simulink model "VCU_SW"  (R2020b)
settings: Solver=FixedStepDiscrete  StartTime=0.0  StopTime=inf  FixedStep=1e-2  RelTol=1e-3
PreLoadFcn:
  | RTWConfigurationCB('preloadfcn', bdroot);
InitFcn:
  | loadvar_ttc500
undefined symbols (not defined in the file): BrkPedalTypes, CabMovModeTypes, cFuseTempSensAcc_X, cFuseTempSensAcc_Y, cFuseTempSensVal_X, cFuseTempSensVal_Y, cTMSTempSensVal_X, cTMSTempSensVal_Y, cTransferCaseSpeedRatio, diag_state, DoorsPositionTypes, dP_filter_Y, DriverOccClassSystemTypes, ErrorValueTypes, fatal_error_callback, IO_ADC_NO_RANGE, LadderStatusTypes, pAnalogCabRotSensAcc, pAnalogCabRotSensMaxVolt, pAnalogCabRotSensMinVolt, pAnalogCabRotSensRange, pAnalogCabRotSensZeroVolt, pBrkActivePress, pCabTiltSensAcc, pCabTiltSensMaxCur, pCabTiltSensMinCur, pDistanceCorrection, pECANManual_BPNEnable, pECANManual_BPNEnabler_Flag, pFilterSensAccRes, pHDirMaxDiffFrq, pHDirSensHighLvl, pHDirSensLowLvl, pMainGearRatio, pMaxFilterSensRes, pMaxFirstPedalSensValue, pMaxFuseTempSensRes, pMaxPressLoss, pMaxPressSensCurrent, pMaxPressValue, pMaxPressValueHydMotAndPump, pMaxPressValueParkDrain, pMaxSecondPedalSensValue, pMaxTempSensVoltage, pMaxTempValue, pMaxTMSTempSensRes, pMinFilterSensRes, pMinFirstPedalSensValue, pMinFuseTempSensRes, pMinPressLoss, pMinPressSensCurrent, pMinPressValue, pMinSecondPedalSensValue, pMinTempSensVoltage, pMinTempValue, pMinTMSTempSensRes, pMotorRingTeethNum, pPedalSensAccuracyPct, pPedalSensAccuracyVolt, pPressLossTreshhold ... (+20)
libraries: TTlibrary x270, canmsglib x127, simulink x88
(part 15 of 17)

== system VCU_SW/InputLayer/InputNetwork/InputCCAN/CCAN100msecProc1/CabMov buttons processing/callTiltFcn/setAutoTiltBut ==
  setAutoTiltBut : TriggerPort  TriggerType=function-call  IsSimulinkFunction=on  FunctionName=setAutoTiltBut  FunctionVisibility=scoped  VariantControl=(inherit)
  Data Store Write1 : DataStoreWrite  DataStoreName=InputFunctionsData  DataStoreElements=InputFunctionsData.stabBut
  Data Store Write2 : DataStoreWrite  DataStoreName=InputFunctionsData  DataStoreElements=InputFunctionsData.returnBut
  Enumerated Constant : simulink/Sources/Enumerated Constant  OutDataTypeStr=Enum: CabMovModeTypes  Value=CabMovModeTypes.CAB_TILT_RETURN  SampleTime=inf
  Enumerated Constant1 : simulink/Sources/Enumerated Constant  OutDataTypeStr=Enum: CabMovModeTypes  Value=CabMovModeTypes.CAB_TILT_STAB  SampleTime=inf
  Enumerated Constant2 : simulink/Sources/Enumerated Constant  OutDataTypeStr=Enum: StateModeTypes  Value=StateModeTypes.STT_DISABLE  SampleTime=inf
  Enumerated Constant3 : simulink/Sources/Enumerated Constant  OutDataTypeStr=Enum: StateModeTypes  Value=StateModeTypes.STT_ENABLE  SampleTime=inf
  Enumerated Constant4 : simulink/Sources/Enumerated Constant  OutDataTypeStr=Enum: StateModeTypes  Value=StateModeTypes.STT_DISABLE  SampleTime=inf
  Enumerated Constant5 : simulink/Sources/Enumerated Constant  OutDataTypeStr=Enum: StateModeTypes  Value=StateModeTypes.STT_ENABLE  SampleTime=inf
  Multiport Switch : MultiPortSwitch  DataPortOrder=Zero-based contiguous  Inputs=2  zeroidx=on
  Multiport Switch1 : MultiPortSwitch  DataPortOrder=Zero-based contiguous  Inputs=2  zeroidx=on
  Relational Operator : RelationalOperator  Operator===  OutDataTypeStr=boolean  RndMeth=Simplest
  Relational Operator1 : RelationalOperator  Operator===  OutDataTypeStr=boolean  RndMeth=Simplest
  state : ArgIn  OutDataTypeStr=Enum: CabMovModeTypes  ArgumentName=state
  wires:
  Multiport Switch1/1 -> Data Store Write1/1
  Enumerated Constant5/1 -> Multiport Switch1/3
  Enumerated Constant4/1 -> Multiport Switch1/2
  Enumerated Constant2/1 -> Multiport Switch/2
  Enumerated Constant3/1 -> Multiport Switch/3
  Multiport Switch/1 -> Data Store Write2/1
  Relational Operator1/1 -> Multiport Switch1/1
  Enumerated Constant1/1 -> Relational Operator1/2
  Relational Operator/1 -> Multiport Switch/1
  Enumerated Constant/1 -> Relational Operator/2
  state/1 -> Relational Operator/1, Relational Operator1/1

== system VCU_SW/InputLayer/InputNetwork/InputCCAN/CCAN100msecProc1/CabMov buttons processing/callTiltFcn/setTiltBut ==
  setTiltBut : TriggerPort  TriggerType=function-call  IsSimulinkFunction=on  FunctionName=setTiltBut  FunctionVisibility=scoped  VariantControl=(inherit)
  Data Store Read1 : DataStoreRead  DataStoreName=InputNetworkData  DataStoreElements=InputNetworkData.CCAN.BJM1.But3CabPitchFwd#InputNetworkData.CCAN.BJM1.But4CabPitchBckwd#InputNetworkData.CCAN.BJM1.But2CabRollLeft#InputNetworkData.CCAN.BJM1.But1CabRollRight
  Data Store Write1 : DataStoreWrite  DataStoreName=InputFunctionsData  DataStoreElements=InputFunctionsData.pitchFwdBut#InputFunctionsData.pitchBckwdBut#InputFunctionsData.rollLeftBut#InputFunctionsData.rollRightBut
  MATLAB Function : MATLAB Function  TreatAsAtomicUnit=on
  state : ArgIn  OutDataTypeStr=Enum: CabMovModeTypes  ArgumentName=state
  wires:
  state/1 -> MATLAB Function/1(state)
  MATLAB Function/1(pitchFwd) -> Data Store Write1/1
  MATLAB Function/2(pitchBckwd) -> Data Store Write1/2
  Data Store Read1/1 -> MATLAB Function/2(FwdBut)
  Data Store Read1/2 -> MATLAB Function/3(BckwdBut)
  Data Store Read1/3 -> MATLAB Function/4(LeftBut)
  Data Store Read1/4 -> MATLAB Function/5(RightBut)
  MATLAB Function/3(rollLeft) -> Data Store Write1/3
  MATLAB Function/4(rollRight) -> Data Store Write1/4

== system VCU_SW/InputLayer/InputNetwork/InputCCAN/CCAN100msecProc1/CabMov buttons processing/callTiltFcn/tiltReturnAchieved ==
  tiltReturnAchieved : TriggerPort  TriggerType=function-call  IsSimulinkFunction=on  FunctionName=tiltReturnAchieved  FunctionVisibility=scoped  VariantControl=(inherit)
  Constant3 : Constant  Value=pTiltAngleThres
  Constant4 : Constant  Value=pTiltAngleThres
  Data Store Read8 : DataStoreRead  DataStoreName=CabineControllerData  DataStoreElements=CabineControllerData.cabRollHullRef
  Data Store Read9 : DataStoreRead  DataStoreName=CabineControllerData  DataStoreElements=CabineControllerData.cabPitchHullRef
  OR3 : Logic  AllPortsSameDT=off  OutDataTypeStr=boolean
  Relational Operator11 : RelationalOperator  Operator=<=  OutDataTypeStr=boolean  RndMeth=Simplest
  Relational Operator9 : RelationalOperator  Operator=<=  OutDataTypeStr=boolean  RndMeth=Simplest
  result : ArgOut  OutDataTypeStr=boolean  ArgumentName=result
  wires:
  Constant3/1 -> Relational Operator9/2
  Data Store Read9/1 -> Relational Operator9/1
  Constant4/1 -> Relational Operator11/2
  OR3/1 -> result/1
  Relational Operator9/1 -> OR3/1
  Relational Operator11/1 -> OR3/2
  Data Store Read8/1 -> Relational Operator11/1

== matlab function VCU_SW/InputLayer/InputNetwork/InputDiagCAN/GetDiagCAN10msec/MATLAB Function ==
  data: ReadUDSmsgFlag output
function  ReadUDSmsgFlag = UDSClientFcn()

persistent flag

serviceSts = getUDSMsgSts(); 
if serviceSts == uint16(0)
    parsingUDSMsg();
    getWriteMsg();
    flag = true;
else
    flag = false;
end

ReadUDSmsgFlag = flag;

end

== matlab function VCU_SW/InputLayer/InputNetwork/InputDiagCAN/GetDiagCAN10msec/Simulink Function2/MATLAB Function2 ==
  data: UDSStruct data_store_memory
function getWriteUdsMsgFcn()

global UDSStruct

persistent flag

if UDSStruct.Service_id == uint8(hex2dec('2E')) && UDSStruct.sucReadFlag == true
    flag = true;
    if UDSStruct.DataIdentifier == uint16(0xB001)
        UDSStruct.TransPumpVolumeMax = uint16(UDSStruct.DataRecord);        
    elseif UDSStruct.DataIdentifier == uint16(0xB002)
        UDSStruct.TransMotorVolumeMin = uint16(UDSStruct.DataRecord);  
    elseif UDSStruct.DataIdentifier == uint16(0xB003)
        UDSStruct.AccelerationPedalMaxEngSpd = uint16(UDSStruct.DataRecord);
    elseif UDSStruct.DataIdentifier == uint16(0xB004)
        UDSStruct.AccelerationPedalMinEngSpd = uint16(UDSStruct.DataRecord);
    elseif UDSStruct.DataIdentifier == uint16(0xB101)
        UDSStruct.EngineSpeedMax = uint16(UDSStruct.DataRecord);
    elseif UDSStruct.DataIdentifier == uint16(0xB102)
        UDSStruct.EngineSpeedMin = uint16(UDSStruct.DataRecord);    
    else
        flag = false; 
    end
else
    flag = false; 
end

UDSStruct.WtiteUDSmsgFlag = flag; 

end

== matlab function VCU_SW/InputLayer/Simulink Function2/MATLAB Function ==
  data: volt input; state output; treshold input
function state = conv(volt, treshold)

if volt > treshold
    state = StateModeTypes.STT_ENABLE;
else
    state = StateModeTypes.STT_DISABLE;
end

end

== matlab function VCU_SW/OutputLayer/OutputNetwork/OutputDiagCAN + Logger/exLogger/MATLAB Function6 ==
  data: input input; value output
function value = fcn(input)

if input == StateModeTypes.STT_DISABLE
    value = uint8(0);
elseif input == StateModeTypes.STT_ENABLE
    value = uint8(1);
else
    value = uint8(0);
end

== matlab function VCU_SW/InputLayer/InputNetwork/InputCCAN/CCAN100msecProc1/CabMov buttons processing/MATLAB Function ==
function buttProcCaller()
    
    rotState = callRotFcn();
    callTiltFcn(rotState);
    
end

== matlab function VCU_SW/OutputLayer/OutputNetwork/OutputDiagCAN + Logger/SetDiagCAN10msec/MATLAB Function ==
  data: flag input
function getUDSmsgFcn(flag)
 
if flag 
    getUDSMsg();
end

end

== matlab function VCU_SW/ServerFcn/convINint1/MATLAB Function2 ==
  data: x input; y output
function y = fcn(x)

y = int16(x);

end

== matlab function VCU_SW/ServerFcn/convAIResistanceData/MATLAB Function ==
  data: inpValue input; outValue output; errorSts input
function outValue = convResValFcn(inpValue, errorSts)

if errorSts == uint16(0)
    %outValue = uint32(inpValue*single(1000));
    outValue = inpValue;
else
    outValue = uint32(ErrorValueTypes.RESISTANSE_ERROR_VALUE);
end

end

== matlab function VCU_SW/InputLayer/InputNetwork/InputCCAN/CCAN100msecProc1/CabMov buttons processing/callRotFcn/RotFcn ==
  data: rotState output; rotReturnTrigger input; manualRotReq input
function rotState = RotFcn(rotReturnTrigger, manualRotReq)

    persistent state
        if isempty(state)
            state = CabMovModeTypes.CAB_FIXED;
            setReturnBut(StateModeTypes.STT_DISABLE);
        end

    switch state
    
        case CabMovModeTypes.CAB_FIXED
            %Первый приоритет - вращение вручную
            if manualRotReq
                state = CabMovModeTypes.CAB_ROTATION;
            elseif rotReturnTrigger && ~rotReturnAchieved()
            %Второй приоритет - автоматический возврат
                state = CabMovModeTypes.CAB_ROTATION_RETURN;
                setReturnBut(StateModeTypes.STT_ENABLE);
            end
            
        case CabMovModeTypes.CAB_ROTATION
            if ~manualRotReq
                state = CabMovModeTypes.CAB_FIXED;
            end
            
        case CabMovModeTypes.CAB_ROTATION_RETURN
            %Выход т.к. джойстик приоритетней
            if manualRotReq
                state = CabMovModeTypes.CAB_ROTATION;
                setReturnBut(StateModeTypes.STT_DISABLE);
            %Выход т.к. закончили возврат либо повторно нажали на кнопку
            elseif rotReturnAchieved() || rotReturnTrigger
                state = CabMovModeTypes.CAB_FIXED;
                setReturnBut(StateModeTypes.STT_DISABLE);
            end
            
    end
        
    rotState = state;
    
end

%bool = rotReturnAchieved() достигнуто целевое положение возврата по
%вращению

%setReturnBut(StateModeTypes) запись в датастор значения кнопки
%автоматического возврата по повороту

%Кнопки с низшим приоритетом не приводят к остановке действия высшего
%приоритета

== matlab function VCU_SW/ServerFcn/convDataStsToEnum/MATLAB Function ==
  data: value input; enum output
function enum = convertToEnumFcn(value)
%#codegen
enum = StatusModeTypes.NO_ACTION;
if value == uint8(0)
    enum = StatusModeTypes.OFF;
elseif value == uint8(1)
    enum = StatusModeTypes.ON;
end
% reserved value is not used yet

end

== matlab function VCU_SW/OutputLayer/OutputNetwork/OutputDiagCAN + Logger/SetDiagCAN10msec/Simulink Function/MATLAB Function1 ==
  data: UDSStruct data_store_memory
function getUDSoutputdata()

global UDSStruct

persistent service_id NRC data_out uds_id_read uds_address_read

if isempty(service_id)
    NRC = uint8(0);
    data_out = uint16(0);
    uds_id_read  = uint16([0x0201 0x0202 0x0203 0x0204 0x0205 0x0206 0x0207 ...
               0x0301 0x0302 0x0303 0x0304 ...
               0x0401 ...
               0x0501 0x0502 0x0503 0x0504 0x0505 0x0506 0x0507 0x0508 0x0509 0x0510 0x0511 ...
               0x0701 0x0702 0x0703 0x0704 0x0705 0x0706 0x0707 0x0708]);  

    uds_address_read  = [UDSStruct.brkFrontCircPressSens UDSStruct.brkRearCircPressSens UDSStruct.brkSupplyFrontPressSens UDSStruct.brkSupplyRearPressSens UDSStruct.brkSupplyParkPressSens UDSStruct.steeringLSPressSens UDSStruct.drainParkPressSens ...
               UDSStruct.cabTiltLeftLongSens UDSStruct.cabTiltLeftTransSens UDSStruct.longitudinalTransPlatfAngleSens UDSStruct.transverseTransPlatfAngleSens ...
               UDSStruct.harvesterHeadPumpPressSens ...
               UDSStruct.hydMotPressLinePressSens UDSStruct.reverseTransmMotPessLinePressSens UDSStruct.hydMotTempSens UDSStruct.transPumpTempSens UDSStruct.transmHydMotSpdSensSig1 UDSStruct.transmHydMotSpdSensSig2 UDSStruct.transmMotDirSens ...
               UDSStruct.transPumpSpdSensSig2 UDSStruct.transPumpSpdSensSig1 UDSStruct.transmPumpDirSens UDSStruct.washerTiltPumpTransSens ...
               UDSStruct.voltageOnT15DO UDSStruct.upperGenWorkSig UDSStruct.lowerGenWorkSig ...
               UDSStruct.driveTransPumpVlv UDSStruct.reverseTransPumpVlv UDSStruct.transMotorVlv UDSStruct.techEquipPumpSupply UDSStruct.strAndBrkPumpDistrSupply];        
end


if UDSStruct.WtiteUDSmsgFlag == true
    service_id = uint8(hex2dec('6E'));
    data_out = uint16(0);
    getPosMess(service_id, UDSStruct.DataIdentifier, data_out);
else
    service_id = uint8(hex2dec('2E'));
    NRC = uint8(hex2dec('31'));
    getNegMess(uint8(hex2dec('7F')), service_id, NRC);
end


if UDSStruct.Service_id == uint8(hex2dec('22'))
    for i=1:length(uds_id_read)
        if UDSStruct.DataIdentifier == uint16(uds_id_read(i))
            service_id = uint8(hex2dec('62'));
            data_out = uint16(uds_address_read(i));
            getPosMess(service_id, UDSStruct.DataIdentifier, data_out);
        else
            service_id = uint8(hex2dec('22'));
            NRC = uint8(hex2dec('31'));
            getNegMess(uint8(hex2dec('7F')), service_id, NRC);
        end
    end
end
    
end

== matlab function VCU_SW/ServerFcn/convUintPinToenumStt/MATLAB Function ==
  data: uintValue input; enum output
function enum = convUintPinToenumSttFcn(uintValue)

if uintValue == uint8(0)
    enum = StateModeTypes.STT_DISABLE;
elseif uintValue == uint8(1)
    enum = StateModeTypes.STT_ENABLE;
elseif uintValue == uint8(2)
    enum = StateModeTypes.STT_ERROR;
else
    enum = StateModeTypes.STT_DEFAULT;
end

end

== matlab function VCU_SW/ServerFcn/convDIOSttToEnum/MATLAB Function ==
  data: value input; enum output; error input
function enum = convertToDIOStsFcn(value, error)
%#codegen
    if error == uint16(0)
        if value
            enum = StateModeTypes.STT_ENABLE;
        else
            enum = StateModeTypes.STT_DISABLE;
        end
    else
        enum = StateModeTypes.STT_ERROR; 
    end
end

== matlab function VCU_SW/InputLayer/InputNetwork/InputCCAN/CCAN100msecProc1/CabMov buttons processing/callTiltFcn/TiltFcn ==
  data: rotState input; stabButTrigger input; tiltReturnTrigger input; tiltPress input
function TiltFcn(rotState, stabButTrigger, tiltReturnTrigger, tiltPress)
  
    monkeyPressAutoTilt = stabButTrigger && tiltReturnTrigger;
    
    persistent state
        if isempty(state)
            state = CabMovModeTypes.CAB_FIXED;
            setAutoTiltBut(state);
        end
        
    if rotState == CabMovModeTypes.CAB_FIXED

        switch state

            case CabMovModeTypes.CAB_FIXED
                if tiltPress %&& ~monkeyPressTilt()
                    state = CabMovModeTypes.CAB_TILT;
                elseif monkeyPressAutoTilt || monkeyPressTilt()
                    %Курим бамбук пока обезьяна не успокоится
                elseif stabButTrigger
                    state = CabMovModeTypes.CAB_TILT_STAB;
                    setAutoTiltBut(state);
                elseif tiltReturnTrigger
                    state = CabMovModeTypes.CAB_TILT_RETURN;
                    setAutoTiltBut(state);
                end

            case CabMovModeTypes.CAB_TILT
                if monkeyPressTilt() || ~tiltPress
                    state = CabMovModeTypes.CAB_FIXED;
                end
                %Если выйдем из состояния, запишутся нули, пока в
                %состоянии, транслируем что приходит
                setTiltBut(state);

            case CabMovModeTypes.CAB_TILT_STAB
                if tiltPress && ~monkeyPressTilt()
                    state = CabMovModeTypes.CAB_TILT;
                    setAutoTiltBut(state);
                elseif monkeyPressAutoTilt || monkeyPressTilt() || stabButTrigger
                    state = CabMovModeTypes.CAB_FIXED;
                    setAutoTiltBut(state);
                elseif tiltReturnTrigger
                    state = CabMovModeTypes.CAB_TILT_RETURN;
                    setAutoTiltBut(state);
                end


            case CabMovModeTypes.CAB_TILT_RETURN
                if tiltPress && ~monkeyPressTilt()
                    state = CabMovModeTypes.CAB_TILT;
                    setAutoTiltBut(state);
                elseif monkeyPressAutoTilt || monkeyPressTilt() ...
                       || tiltReturnTrigger || tiltReturnAchieved()
                    state = CabMovModeTypes.CAB_FIXED;
                    setAutoTiltBut(state);
                elseif stabButTrigger
                    state = CabMovModeTypes.CAB_TILT_STAB;
                    setAutoTiltBut(state);
                end
        end
        
    elseif state ~= CabMovModeTypes.CAB_FIXED
        state = CabMovModeTypes.CAB_FIXED;
        setAutoTiltBut(state);
        setTiltBut(state);
    end
        
    
end

%setAutoTiltBut(state); по возvожным режимам (CAB_TILT_STAB,
%CAB_TILT_RETURN, другое) записывает в датастор нужную кнопку, отжимая другие

%setTiltBut(state) пишет в кнопки наклона нули, если state не CAB_TILT,
%иначе текущую кнопку наклона

%bool = monkeyPressTilt() нажато больше одной кнопки ручного наклона

%bool = tiltPress() активна любая кнопка ручного наклона

%bool = stabButTrigger(); нажата кнопка стабилизации

%bool = tiltReturnButTrigger() нажата кнопка автоматического возврата по
%наклону(триггер)

%bool = tiltReturnAchieved() достигли вертикального положения отн. рамы

%Кнопки с низшим приоритетом не приводят к остановке действия высшего
%приоритета

== matlab function VCU_SW/ServerFcn/convAIVoltageData/MATLAB Function ==
  data: inpValue input; outValue output; errorSts input
function outValue = convVoltValFcn(inpValue, errorSts)
%convert to mV if input data in μV!
if errorSts == uint16(0)
    %outValue = uint16(inpValue*single(1000));
    outValue = uint16(inpValue);
else
    outValue = uint16(ErrorValueTypes.VOLTAGE_ERROR_VALUE);
end


end

== matlab function VCU_SW/InputLayer/InputNetwork/InputCCAN/CCAN100msecProc1/CabMov buttons processing/callTiltFcn/setTiltBut/MATLAB Function ==
  data: state input; pitchFwd output; FwdBut input; BckwdBut input; LeftBut input; RightBut input; pitchBckwd output; rollLeft output; rollRight output
function [pitchFwd, pitchBckwd, rollLeft, rollRight] = setButtons(state, FwdBut, BckwdBut, LeftBut, RightBut)

if state == CabMovModeTypes.CAB_TILT
    pitchFwd = FwdBut;
    pitchBckwd = BckwdBut;
    rollLeft = LeftBut;
    rollRight = RightBut;
else
    pitchFwd = StateModeTypes.STT_DISABLE;
    pitchBckwd = StateModeTypes.STT_DISABLE;
    rollLeft = StateModeTypes.STT_DISABLE;
    rollRight = StateModeTypes.STT_DISABLE;
end

end

== matlab function VCU_SW/ServerFcn/convAICurrentData/MATLAB Function ==
  data: inpValue input; outValue output; errorSts input
function outValue = convCurValFcn(inpValue, errorSts)
%convert to mA if input data in μA!
if errorSts == uint16(0)
    %outValue = uint16(inpValue/single(1000));
    outValue = uint16(inpValue);
else
    outValue = uint16(ErrorValueTypes.CURRENT_ERROR_VALUE);
end

end

== matlab function VCU_SW/ServerFcn/calcCRC16/MATLAB Function ==
  data: packet input; crcfinal output
function crcfinal = crc16_3(packet)

    crc = uint16(0);
    for i = 1:length(packet)
        %reverse bits in byte
        byte = uint16(0);
        high = uint16(hex2dec('0080'));
        low = uint16(hex2dec('0001'));
        while high ~= uint16(0)
            if uint8(bitand(packet(i), high)) > uint8(0)
                byte = bitxor(byte, low);
            end
            high = bitshift(high, -1);
            low = bitshift(low, 1);
        end
        %byte processing
        crc = bitxor(crc, bitshift(byte,8) );
        for bit = 1:8
            if bitand( crc, hex2dec('8000') )  
              crc = bitxor( bitshift(crc,1), hex2dec('C86C') );
            else
              crc = bitshift(crc,1);
            end
            crc = bitand( crc, hex2dec('FFFF') );  % trim to 16 bits
        end
    end
    %reverse bits in crc
    crcfinal = uint16(0);
    high = uint16(hex2dec('8000'));
    low = uint16(hex2dec('0001'));
    while high ~= uint16(0)
        if uint8(bitand(crc, high)) > uint8(0)
            crcfinal = bitxor(crcfinal, low);
        end
        high = bitshift(high, -1);
        low = bitshift(low, 1);
    end  
end

== matlab function VCU_SW/ServerFcn/convPWDData/MATLAB Function ==
  data: inpValue input; outValue output; errorSts input
function outValue = convResValFcn(inpValue, errorSts)

if errorSts == uint16(0)
    outValue = uint16(inpValue/uint32(1000));
else
    outValue = uint16(ErrorValueTypes.FREQ_ERROR_VALUE);
end

end

== matlab function VCU_SW/ServerFcn/convDIOStsTypeToNum/MATLAB Function ==
  data: enum input; value output
function value = convertDIOStsToNumFcn(enum)
%#codegen
    if enum == StateModeTypes.STT_ENABLE
        value = true;
    else
        value = false;
    end
% for future, if there is error or warning, then set function is not called
end

== matlab function VCU_SW/ServerFcn/calcMaxVal/MATLAB Function ==
  data: fstValue input; maxValue output; secValue input
function maxValue = maxFcn(fstValue, secValue)
%#codegen
%because fuck matlab, that's why
%
%     if fstValue > secValue
%         maxValue = fstValue;
%     else
%         maxValue = secValue;
%     end
% i must to create magic function, because previous code matlab compilier
% generate, like standart fcn - fabsf a i catch error
%     if abs(fstValue - secValue) < single(0.001)
%         maxValue = fstValue;
%     elseif fstValue > secValue
%         maxValue = fstValue;
%     else
%         maxValue = secValue;
%     end
% the same...
end

== matlab function VCU_SW/InputLayer/InputInterfaces/PWMCurrentInput/PWMCur10msecProc/MATLAB Function2 ==
  data: sttRaw input; sttInv output
function sttInv = invert(sttRaw)
    
    if sttRaw == StateModeTypes.STT_ENABLE
        sttInv = StateModeTypes.STT_DISABLE;
    elseif sttRaw == StateModeTypes.STT_DISABLE
        sttInv = StateModeTypes.STT_ENABLE;
    else
        sttInv = sttRaw;
    end
    
end

== matlab function VCU_SW/InputLayer/InputNetwork/InputCCAN/GetCCAN100msec/CabinAuxiliaryStatus/MATLAB Function ==
  data: Value input; LadderStatus output
function LadderStatus = calcLadderStatus(Value)
    
    if Value == uint8(0)
        LadderStatus = LadderStatusTypes.LADDER_UP;
    elseif Value == uint8(1)
        LadderStatus = LadderStatusTypes.LADDER_DOWN;
    elseif Value == uint8(2)
        LadderStatus = LadderStatusTypes.LADDER_RESERVED;
    else
        LadderStatus = LadderStatusTypes.LADDER_NOT_AVAILABLE;
    end
end

== matlab function VCU_SW/ServerFcn/calcMinVal/MATLAB Function ==
  data: fstValue input; minValue output; secValue input
function minValue = minFcn(fstValue, secValue)
%#codegen
%because fuck matlab, that's why
    if fstValue < secValue
        minValue = fstValue;
    else
        minValue = secValue;
    end
end

== matlab function VCU_SW/InputLayer/InputInterfaces/DigitalInput/Function-Call Subsystem2/MATLAB Function ==
  data: sensSupply1 input; sensSupply2 input
  events: fcncall output FUNCTION_CALL_EVENT
function fcn(sensSupply1, sensSupply2)

    persistent timer
        if isempty(timer)
            timer = uint8(0);
        end
        
    if sensSupply1 == StateModeTypes.STT_ENABLE && sensSupply2 == StateModeTypes.STT_ENABLE
        if timer < uint8(1000)
            timer = timer + uint8(1);
        end
    end
    
    if timer >= uint8(1000)
        fcncall();
    end
    
end

== matlab function VCU_SW/InputLayer/InputInterfaces/DigitalInput/Function-Call Subsystem2/cabRotIndSensProc/cabRotIndSensProc fcn ==
  data: pResetIndCabSensErr input
function cabRotIndSensProc(pResetIndCabSensErr)
    
    persistent err
    if isempty(err)
        err = false;
    end
    
    if err
        if pResetIndCabSensErr
            err = false;
            setIndSensErr(err);
        end        
    else
        cabRotPos = getIndRotSensData();
        if cabRotPos == CabRotPosTypes.ROTPOS_ERROR
            err = true;
            setIndSensErr(err);
        else
            setIndRotSensData(cabRotPos);
        end        
    end

end

== matlab function VCU_SW/InputLayer/InputInterfaces/DigitalInput/Function-Call Subsystem2/cabRotIndSensProc/getIndRotSensData/getIndRotSensData fcn ==
  data: cabPos output; indSensRight input
function cabPos = getIndRotSensData(indSensRight)

    if indSensRight == StateModeTypes.STT_ENABLE 
        cabPos = CabRotPosTypes.ROTPOS_NEAR_ZERO;
    elseif (indSensRight == StateModeTypes.STT_DISABLE)&&...
           (indSensLeft == StateModeTypes.STT_ENABLE)
        cabPos = CabRotPosTypes.ROTPOS_LEFT;
    elseif (indSensRight == StateModeTypes.STT_ENABLE)&&...
           (indSensLeft == StateModeTypes.STT_DISABLE)
        cabPos = CabRotPosTypes.ROTPOS_RIGHT;
    elseif (indSensRight == StateModeTypes.STT_DISABLE)&&...
           (indSensLeft == StateModeTypes.STT_DISABLE)
        switch getRotPos()
            case {CabRotPosTypes.ROTPOS_LEFT, CabRotPosTypes.ROTPOS_LEFT_END}
                cabPos = CabRotPosTypes.ROTPOS_LEFT_END;
            case {CabRotPosTypes.ROTPOS_RIGHT, CabRotPosTypes.ROTPOS_RIGHT_END}
                cabPos = CabRotPosTypes.ROTPOS_RIGHT_END;
            otherwise
                cabPos = CabRotPosTypes.ROTPOS_ERROR;
        end    
    else
        cabPos = CabRotPosTypes.ROTPOS_ERROR;
    end
    
end

== matlab function VCU_SW/ServerFcn/convDiagDataForTest/MATLAB Function ==
  data: hwDiag input; canDiag output
function canDiag = fcn(hwDiag)

if hwDiag == uint16(0)
    canDiag = uint8(0);
elseif hwDiag == uint16(10)
    canDiag = uint8(1);
elseif hwDiag == uint16(11)
    canDiag = uint8(3);
elseif hwDiag == uint16(12)
    canDiag = uint8(2);
elseif hwDiag == uint16(13)
    canDiag = uint8(4);
else
    canDiag = uint8(5);
end




end

== matlab function VCU_SW/ServerFcn/convDIOSttTypeToNum/MATLAB Function ==
  data: enum input; value output
function value = convertDIOStsToNumFcn(enum)
%#codegen
if enum == StateModeTypes.STT_DISABLE
    value = uint8(0);
elseif enum == StateModeTypes.STT_ENABLE
    value = uint8(1);
elseif enum == StateModeTypes.STT_ERROR
    value = uint8(2);
else
    value = uint8(3);
end

end

== matlab function VCU_SW/ServerFcn/calcAbsVal/MATLAB Function ==
  data: fstValue input; minValue output; secValue input
function minValue = minFcn(fstValue, secValue)
%#codegen
%because fuck matlab, that's why
    if fstValue < secValue
        minValue = fstValue;
    else
        minValue = secValue;
    end
end

== matlab function VCU_SW/EEPROM Layer/EEPROM Client ==
  data: t15common input; sucReadFlag output; sucWriteFlag output
function [sucReadFlag, sucWriteFlag] = EEPROMControl( t15common )

    persistent data_read_successful data_write_successful t15common_old read_reqest write_reqest
        if isempty(data_read_successful)
            data_read_successful = false;
            data_write_successful = false;
            t15common_old = StateModeTypes.STT_DISABLE;
            read_reqest = false;
            write_reqest = false;
        end
    
    %Вынести в инпут
    if t15common == StateModeTypes.STT_ENABLE ...
       && data_read_successful
        updateUDSStruct();
    end
    
    %Запрос на запись при включении T15
    if t15common_old == StateModeTypes.STT_DISABLE ...
       && t15common == StateModeTypes.STT_ENABLE
        read_reqest = true;
    %Запрос на чтение при отключении T15    
    elseif t15common_old == StateModeTypes.STT_ENABLE ...
           && t15common == StateModeTypes.STT_DISABLE
        write_reqest = true;
    end
    
    %Выполняется до тех пор, пока есть запрос и не событие произошло успешно
    if ~data_read_successful && read_reqest == true
        data_read_successful = readProcessing();
    end
    
    if data_read_successful ...
       && ~data_write_successful ...
       && write_reqest == true
        data_write_successful = writeProcessing();
    end
    
    t15common_old = t15common;
    
    sucReadFlag = data_read_successful;
    sucWriteFlag = data_write_successful;
    
end
% global EEPROMData
% persistent cnt exT15state rst_cnt
% if isempty(cnt)
%     cnt = uint8(0);
%     exT15state = t15common;
%     rst_cnt = uint8(0);
% end
% 
% if EEPROMData.alreadyReadFlag ~= StateModeTypes.STT_ENABLE
%     readDistance();
% end
% 
% if t15common ~= StateModeTypes.STT_ENABLE && exT15state == StateModeTypes.STT_ENABLE
%     EEPROMData.writingInProcessFl = StateModeTypes.STT_ENABLE;
% end
% 
% if EEPROMData.writingInProcessFl == StateModeTypes.STT_ENABLE && cnt < uint8(50)
%     cnt = cnt + uint8(1);
% else
%     EEPROMData.writingInProcessFl = StateModeTypes.STT_DISABLE;
%     if cnt ~= uint8(0)
%         cnt = uint8(0);
%     end
% end
% 
% if EEPROMData.writingInProcessFl == StateModeTypes.STT_ENABLE
%     if cnt == uint8(15)
%         if EEPROMData.updatedDistM ~= EEPROMData.savedDistM
%             write();
%         end
%     end
% 
%     if cnt == uint8(48)
%          EEPROMData.tripDistM = uint32(0);
%     end
% end
% 
% if tripReset == uint8(1)
%     
%     if rst_cnt < uint8(200)
%         
%         rst_cnt = rst_cnt + uint8(1);
%         
%     else
%        
%         if EEPROMData.Trip_Reset ~= StateModeTypes.STT_ENABLE
%             
%             EEPROMData.Trip_Reset = StateModeTypes.STT_ENABLE;
%             
%         end
%         
%     end
%     
% else
%     
%     if rst_cnt > uint8(0)
%         
%         rst_cnt = uint8(0);
%         
%     end
%     
%     if EEPROMData.Trip_Reset ~= StateModeTypes.STT_DISABLE
%         
%         EEPROMData.Trip_Reset = StateModeTypes.STT_DISABLE;
%         
%     end
%     
% end
% 
% exT15state = t15common;

== matlab function VCU_SW/EEPROM Layer/Simulink Function3/eeprom_write_processing_kora ==
  data: UDSStruct data_store_memory; eeprom_sts output
function eeprom_sts  = get_eeprom_status
    
    eeprom_sts_local = uint16(15);

    if (coder.target('MATLAB')) || (coder.target('Sfun'))

    else
        
        eeprom_sts_local = coder.ceval('get_eeprom_status');
         
    end
    
    eeprom_sts = eeprom_sts_local;
    
end

== matlab function VCU_SW/EEPROM Layer/readProcessing/eeprom_read_processing_kora ==
  data: UDSStruct data_store_memory; flag output
function flag = readProcessing()

    global UDSStruct
    
    %Флаг успешной записи в структуру
    flag = false;
    
    if (coder.target('MATLAB')) || (coder.target('Sfun'))

    else
        %Получение флага успешного чтения из EEPROM
        read_flag = uint8(0);
        read_flag = coder.ceval('get_read_flag');
        
        %Получение даных после второго успешного чтения
        %Первое успешное чтение обман (с) Ваня
        if read_flag == 2

            data = zeros(10, 1, 'uint32');
            coder.ceval('get_EEPROM_data', data);

            UDSStruct.TotalDistance = uint32(data(1));
            UDSStruct.TotalEngineHours = uint32(data(2));
            UDSStruct.TransPumpVolumeMax = uint16(data(3));
            UDSStruct.TransMotorVolumeMin = uint16(data(4));
            UDSStruct.AccelerationPedalMaxEngSpd = uint16(data(5));
            UDSStruct.AccelerationPedalMinEngSpd = uint16(data(6));
            UDSStruct.EngineSpeedMax = uint16(data(7));
            UDSStruct.EngineSpeedMin = uint16(data(8));
            
            flag = true;
            
        end
        
    end
    
end

== matlab function VCU_SW/EEPROM Layer/writeProcessing/eeprom_write_processing_kora ==
  data: UDSStruct data_store_memory; flag output
function flag = writeProcessing()

    global UDSStruct
    
    %флаг вызова фунцкии записи
    flag = false;
    
    if (coder.target('MATLAB')) || (coder.target('Sfun'))

    else
        
        data = zeros(9, 1, 'uint32');
        data(1) = uint32(UDSStruct.TotalDistance);
        data(2) = uint32(UDSStruct.TotalEngineHours);
        data(3) = uint32(UDSStruct.TransPumpVolumeMax);
        data(4) = uint32(UDSStruct.TransMotorVolumeMin);
        data(5) = uint32(UDSStruct.AccelerationPedalMaxEngSpd);
        data(6) = uint32(UDSStruct.AccelerationPedalMinEngSpd);
        data(7) = uint32(UDSStruct.EngineSpeedMax);
        data(8) = uint32(UDSStruct.EngineSpeedMin);
        
        %Вызов функции перекладывания данных в буфер EEPROM
        coder.ceval('put_EEPROM_data', data);
        %Выставление флага записи в буфер
        coder.ceval('set_write_flag', uint8(1));
                
        flag = true;
        
    end
    
end

== matlab function VCU_SW/InputLayer/InputNetwork/InputDiagCAN/GetDiagCAN10msec1/MATLAB Function ==
  data: UDSStruct data_store_memory
function UDSClientFcn

global UDSStruct

parsingUDSMsg();
if UDSStruct.readUDSmsgFlag
    getWriteMsg();
end
end

== matlab function VCU_SW/InputLayer/InputNetwork/InputDiagCAN/GetDiagCAN10msec1/Simulink Function2/MATLAB Function2 ==
  data: UDSStruct data_store_memory
function getWriteUdsMsgFcn()

global UDSStruct

if UDSStruct.Service_id == uint8(0x2E)
    if UDSStruct.DataIdentifier == uint16(0xB001)
        UDSStruct.TransPumpVolumeMax = uint16(UDSStruct.DataRecord);        
    elseif UDSStruct.DataIdentifier == uint16(0xB002)
        UDSStruct.TransMotorVolumeMin = uint16(UDSStruct.DataRecord);  
    elseif UDSStruct.DataIdentifier == uint16(0xB003)
        UDSStruct.AccelerationPedalMaxEngSpd = uint16(UDSStruct.DataRecord);
    elseif UDSStruct.DataIdentifier == uint16(0xB004)
        UDSStruct.AccelerationPedalMinEngSpd = uint16(UDSStruct.DataRecord);
    elseif UDSStruct.DataIdentifier == uint16(0xB101)
        UDSStruct.EngineSpeedMax = uint16(UDSStruct.DataRecord);
    elseif UDSStruct.DataIdentifier == uint16(0xB102)
        UDSStruct.EngineSpeedMin = uint16(UDSStruct.DataRecord);     
    end
end
end

== matlab function VCU_SW/OutputLayer/OutputNetwork/OutputDiagCAN + Logger/SetDiagCAN10msec1/MATLAB Function ==
  data: readflag input
function getUDSmsgFcn(readflag)

if readflag
    getUDSMsg();
end

end

== matlab function VCU_SW/InputLayer/InputNetwork/InputDiagCAN/GetDiagCAN10msec1/Simulink Function1/MATLAB Function ==
  data: errSts input; ReadUDSmsgFlag output
function ReadUDSmsgFlag = fcn(errSts)

persistent flag

if errSts == uint8(0)
flag = uint8(1);
else
flag = uint8(0);
end


ReadUDSmsgFlag = flag;

end

== matlab function VCU_SW/OutputLayer/OutputNetwork/OutputDiagCAN + Logger/SetDiagCAN10msec1/Simulink Function/MATLAB Function1 ==
  data: UDSStruct data_store_memory
function getUDSoutputdata()

global UDSStruct

if UDSStruct.Service_id == uint8(0x2E) || UDSStruct.Service_id == uint8(0x22)
    switch UDSStruct.DataIdentifier
       case uint16(0xB001)
           if UDSStruct.Service_id == uint8(0x2E)
                getPosMess(uint8(0x6E), UDSStruct.DataIdentifier, uint16(0));
           elseif UDSStruct.Service_id == uint8(0x22)
                getPosMess(uint8(0x62), UDSStruct.DataIdentifier, uint16(UDSStruct.TransPumpVolumeMax));
           end
       case uint16(0xB002)
           if UDSStruct.Service_id == uint8(0x2E)
                getPosMess(uint8(0x6E), UDSStruct.DataIdentifier, uint16(0));
           elseif UDSStruct.Service_id == uint8(0x22)
                getPosMess(uint8(0x62), UDSStruct.DataIdentifier, uint16(UDSStruct.TransMotorVolumeMin));
           end
       case uint16(0xB003)
           if UDSStruct.Service_id == uint8(0x2E)
                getPosMess(uint8(0x6E), UDSStruct.DataIdentifier, uint16(0));
           elseif UDSStruct.Service_id == uint8(0x22)
                getPosMess(uint8(0x62), UDSStruct.DataIdentifier, uint16(UDSStruct.AccelerationPedalMaxEngSpd));
           end
       case uint16(0xB004)
           if UDSStruct.Service_id == uint8(0x2E)
                getPosMess(uint8(0x6E), UDSStruct.DataIdentifier, uint16(0));
           elseif UDSStruct.Service_id == uint8(0x22)
                getPosMess(uint8(0x62), UDSStruct.DataIdentifier, uint16(UDSStruct.AccelerationPedalMinEngSpd));
           end
       case uint16(0xB101)
           if UDSStruct.Service_id == uint8(0x2E)
                getPosMess(uint8(0x6E), UDSStruct.DataIdentifier, uint16(0));
           elseif UDSStruct.Service_id == uint8(0x22)
                getPosMess(uint8(0x62), UDSStruct.DataIdentifier, uint16(UDSStruct.EngineSpeedMax));
           end
       case uint16(0xB102)
           if UDSStruct.Service_id == uint8(0x2E)
                getPosMess(uint8(0x6E), UDSStruct.DataIdentifier, uint16(0));
           elseif UDSStruct.Service_id == uint8(0x22)
                getPosMess(uint8(0x62), UDSStruct.DataIdentifier, uint16(UDSStruct.EngineSpeedMin));
           end

       case uint16(0x0709)
          getPosMess(uint8(0x62), UDSStruct.DataIdentifier, uint16(UDSStruct.pin_transCaseHighGearIsActiveSens));
       case uint16(0x070A)
          getPosMess(uint8(0x62), UDSStruct.DataIdentifier, uint16(UDSStruct.pin_transCaseLowGearIsActiveSens));
       case uint16(0x070B)
          getPosMess(uint8(0x62), UDSStruct.DataIdentifier, uint16(UDSStruct.pin_lowBrkFluidLvlSens));
       case uint16(0x070C)
          getPosMess(uint8(0x62), UDSStruct.DataIdentifier, uint16(UDSStruct.pin_T15Common));
       case uint16(0x070D)
          getPosMess(uint8(0x62), UDSStruct.DataIdentifier, uint16(UDSStruct.pin_lowCenLubrOilLvl));
       case uint16(0x070E)
          getPosMess(uint8(0x62), UDSStruct.DataIdentifier, uint16(UDSStruct.pin_shutdownButtonSig));      
       case uint16(0x070F)
          getPosMess(uint8(0x62), UDSStruct.DataIdentifier, uint16(UDSStruct.pin_stopLightsSens));      
       case uint16(0x0710)
          getPosMess(uint8(0x62), UDSStruct.DataIdentifier, uint16(UDSStruct.pin_TermACC_Supply));
       case uint16(0x0711)
          getPosMess(uint8(0x62), UDSStruct.DataIdentifier, uint16(UDSStruct.pin_T50_Supply)); 
       case uint16(0x0712)
          getPosMess(uint8(0x62), UDSStruct.DataIdentifier, uint16(UDSStruct.pin_engAirFilterClogSens)); 
       case uint16(0x0713)
          getPosMess(uint8(0x62), UDSStruct.DataIdentifier, uint16(UDSStruct.pin_selector_signal_1));
       case uint16(0x0714)
          getPosMess(uint8(0x62), UDSStruct.DataIdentifier, uint16(UDSStruct.pin_selector_signal_2));
       case uint16(0x0715)
          getPosMess(uint8(0x62), UDSStruct.DataIdentifier, uint16(UDSStruct.pin_selector_signal_3));
       case uint16(0x0716)
          getPosMess(uint8(0x62), UDSStruct.DataIdentifier, uint16(UDSStruct.pin_extrLeftCabPosSens));
       case uint16(0x0717)
          getPosMess(uint8(0x62), UDSStruct.DataIdentifier, uint16(UDSStruct.pin_extrRightCabPosSens));
       case uint16(0x0718)
          getPosMess(uint8(0x62), UDSStruct.DataIdentifier, uint16(UDSStruct.pin_temporaryButton));      
       case uint16(0x0719)
          getPosMess(uint8(0x62), UDSStruct.DataIdentifier, uint16(UDSStruct.pin_transmHydMotSpdSensSig1));      
       case uint16(0x071A)
          getPosMess(uint8(0x62), UDSStruct.DataIdentifier, uint16(UDSStruct.pin_transmHydMotSpdSensSig2));
       case uint16(0x071B)
          getPosMess(uint8(0x62), UDSStruct.DataIdentifier, uint16(UDSStruct.pin_transPumpSpdSensSig2)); 
       case uint16(0x071C)
          getPosMess(uint8(0x62), UDSStruct.DataIdentifier, uint16(UDSStruct.pin_transPumpSpdSensSig1)); 
       case uint16(0x071D)
          getPosMess(uint8(0x62), UDSStruct.DataIdentifier, uint16(UDSStruct.pin_accPedSens1));
       case uint16(0x071E)
          getPosMess(uint8(0x62), UDSStruct.DataIdentifier, uint16(UDSStruct.pin_accPedSens2));
       case uint16(0x071F)
          getPosMess(uint8(0x62), UDSStruct.DataIdentifier, uint16(UDSStruct.pin_filterClogSens));
       case uint16(0x0720)
          getPosMess(uint8(0x62), UDSStruct.DataIdentifier, uint16(UDSStruct.pin_hydMotPressLinePressSens));
       case uint16(0x0721)
          getPosMess(uint8(0x62), UDSStruct.DataIdentifier, uint16(UDSStruct.pin_rotCabAngleSens1));
       case uint16(0x0722)
          getPosMess(uint8(0x62), UDSStruct.DataIdentifier, uint16(UDSStruct.pin_rotCabAngleSens2));      
       case uint16(0x0723)
          getPosMess(uint8(0x62), UDSStruct.DataIdentifier, uint16(UDSStruct.pin_longitudinalTransPlatfAngleSens));      
       case uint16(0x0724)
          getPosMess(uint8(0x62), UDSStruct.DataIdentifier, uint16(UDSStruct.pin_transverseTransPlatfAngleSens));
       case uint16(0x0725)
          getPosMess(uint8(0x62), UDSStruct.DataIdentifier, uint16(UDSStruct.pin_harvesterHeadPumpPressSens)); 
       case uint16(0x0726)
          getPosMess(uint8(0x62), UDSStruct.DataIdentifier, uint16(UDSStruct.pin_brkRearCircPressSens)); 
       case uint16(0x0727)
          getPosMess(uint8(0x62), UDSStruct.DataIdentifier, uint16(UDSStruct.pin_brkFrontCircPressSens));
       case uint16(0x0728)
          getPosMess(uint8(0x62), UDSStruct.DataIdentifier, uint16(UDSStruct.pin_hydMotTempSens));
       case uint16(0x0729)
          getPosMess(uint8(0x62), UDSStruct.DataIdentifier, uint16(UDSStruct.pin_brkSupplyRearPressSens));
       case uint16(0x072A)
          getPosMess(uint8(0x62), UDSStruct.DataIdentifier, uint16(UDSStruct.pin_brkSupplyFrontPressSens));
       case uint16(0x072B)
          getPosMess(uint8(0x62), UDSStruct.DataIdentifier, uint16(UDSStruct.pin_brkSupplyParkPressSens));
       case uint16(0x072C)
          getPosMess(uint8(0x62), UDSStruct.DataIdentifier, uint16(UDSStruct.pin_steeringLSPressSens));      
       case uint16(0x072D)
          getPosMess(uint8(0x62), UDSStruct.DataIdentifier, uint16(UDSStruct.pin_transmPumpDirSens));      
       case uint16(0x072E)
          getPosMess(uint8(0x62), UDSStruct.DataIdentifier, uint16(UDSStruct.pin_transmMotDirSens));
       case uint16(0x072F)
          getPosMess(uint8(0x62), UDSStruct.DataIdentifier, uint16(UDSStruct.pin_washerTiltPumpTransSens)); 
       case uint16(0x0730)
          getPosMess(uint8(0x62), UDSStruct.DataIdentifier, uint16(UDSStruct.pin_reverseTransmMotPessLinePressSens));    
       case uint16(0x0731)
          getPosMess(uint8(0x62), UDSStruct.DataIdentifier, uint16(UDSStruct.pin_cabTiltLeftLongSens));      
       case uint16(0x0732)
          getPosMess(uint8(0x62), UDSStruct.DataIdentifier, uint16(UDSStruct.pin_transPumpTempSens));      
       case uint16(0x0733)
          getPosMess(uint8(0x62), UDSStruct.DataIdentifier, uint16(UDSStruct.pin_drainParkPressSens));
       case uint16(0x0734)
          getPosMess(uint8(0x62), UDSStruct.DataIdentifier, uint16(UDSStruct.pin_voltageOnT15DO)); 
       case uint16(0x0735)
          getPosMess(uint8(0x62), UDSStruct.DataIdentifier, uint16(UDSStruct.pin_upperGenWorkSig));  
       case uint16(0x0736)
          getPosMess(uint8(0x62), UDSStruct.DataIdentifier, uint16(UDSStruct.pin_lowerGenWorkSig)); 
       case uint16(0x0737)
          getPosMess(uint8(0x62), UDSStruct.DataIdentifier, uint16(UDSStruct.pin_HydCANPowerSupply));
       case uint16(0x0738)
          getPosMess(uint8(0x62), UDSStruct.DataIdentifier, uint16(UDSStruct.pin_T15_Supply));
       case uint16(0x0739)
          getPosMess(uint8(0x62), UDSStruct.DataIdentifier, uint16(UDSStruct.pin_IgnitionSwitchPowerSupply));
       case uint16(0x073A)
          getPosMess(uint8(0x62), UDSStruct.DataIdentifier, uint16(UDSStruct.pin_engAirFilterClogSensSupply));
       case uint16(0x073B)
          getPosMess(uint8(0x62), UDSStruct.DataIdentifier, uint16(UDSStruct.pin_extrLeftCabPosSensSupply));
       case uint16(0x073C)
          getPosMess(uint8(0x62), UDSStruct.DataIdentifier, uint16(UDSStruct.pin_extrRightCabPosSensSupply));      
       case uint16(0x073D)
          getPosMess(uint8(0x62), UDSStruct.DataIdentifier, uint16(UDSStruct.pin_transCaseSensSupply));      
       case uint16(0x073E)
          getPosMess(uint8(0x62), UDSStruct.DataIdentifier, uint16(UDSStruct.pin_transPumpPressLinesPressSensSupply));
       case uint16(0x073F)
          getPosMess(uint8(0x62), UDSStruct.DataIdentifier, uint16(UDSStruct.pin_upperGenT15)); 
       case uint16(0x0740)
          getPosMess(uint8(0x62), UDSStruct.DataIdentifier, uint16(UDSStruct.pin_brkSensSupply));    
       case uint16(0x0741)
          getPosMess(uint8(0x62), UDSStruct.DataIdentifier, uint16(UDSStruct.pin_rearAxleDifSupply));      
       case uint16(0x0742)
          getPosMess(uint8(0x62), UDSStruct.DataIdentifier, uint16(UDSStruct.pin_frontAxleDifSupply));      
       case uint16(0x0743)
          getPosMess(uint8(0x62), UDSStruct.DataIdentifier, uint16(UDSStruct.pin_lowerGenT15));
       case uint16(0x0744)
          getPosMess(uint8(0x62), UDSStruct.DataIdentifier, uint16(UDSStruct.pin_diagLamp)); 
       case uint16(0x0745)
          getPosMess(uint8(0x62), UDSStruct.DataIdentifier, uint16(UDSStruct.pin_lowerGearDistrTCSupply));  
       case uint16(0x0746)
          getPosMess(uint8(0x62), UDSStruct.DataIdentifier, uint16(UDSStruct.pin_upperGearDistrTCSupply));      
       case uint16(0x0747)
          getPosMess(uint8(0x62), UDSStruct.DataIdentifier, uint16(UDSStruct.pin_disablingFrontDrDistrSupply));
       case uint16(0x0748)
          getPosMess(uint8(0x62), UDSStruct.DataIdentifier, uint16(UDSStruct.pin_starterSolenoidCtrl));
       case uint16(0x0749)
          getPosMess(uint8(0x62), UDSStruct.DataIdentifier, uint16(UDSStruct.pin_techEquipPumpPressSensSupply));
       case uint16(0x074A)
          getPosMess(uint8(0x62), UDSStruct.DataIdentifier, uint16(UDSStruct.pin_lowBrakeFluidSensSupply));
       case uint16(0x074B)
          getPosMess(uint8(0x62), UDSStruct.DataIdentifier, uint16(UDSStruct.pin_frontBrkDistrLSSupply));      
       case uint16(0x074C)
          getPosMess(uint8(0x62), UDSStruct.DataIdentifier, uint16(UDSStruct.pin_parkBrkDistrLSSupply));      
       case uint16(0x074D)
          getPosMess(uint8(0x62), UDSStruct.DataIdentifier, uint16(UDSStruct.pin_steeringDistrSupply));      
       case uint16(0x074E)
          getPosMess(uint8(0x62), UDSStruct.DataIdentifier, uint16(UDSStruct.pin_parkBrkDistrSupply));
       case uint16(0x074F)
          getPosMess(uint8(0x62), UDSStruct.DataIdentifier, uint16(UDSStruct.pin_rearBrkDistrLSSupply)); 
       case uint16(0x0750)
          getPosMess(uint8(0x62), UDSStruct.DataIdentifier, uint16(UDSStruct.pin_stopLightSensSupply));          
       case uint16(0x0751)
          getPosMess(uint8(0x62), UDSStruct.DataIdentifier, uint16(UDSStruct.pin_strAndBrkPumpDistrSensSupply));      
       case uint16(0x0752)
          getPosMess(uint8(0x62), UDSStruct.DataIdentifier, uint16(UDSStruct.pin_cabRotBlockVlvSupply));      
       case uint16(0x0753)
          getPosMess(uint8(0x62), UDSStruct.DataIdentifier, uint16(UDSStruct.pin_engPreheaterActivationSig));
       case uint16(0x0754)
          getPosMess(uint8(0x62), UDSStruct.DataIdentifier, uint16(UDSStruct.pin_cabAndPlatformTiltSensSupply)); 
       case uint16(0x0755)
          getPosMess(uint8(0x62), UDSStruct.DataIdentifier, uint16(UDSStruct.pin_brkSupplyCircPressSensSupply)); 
       case uint16(0x0756)
          getPosMess(uint8(0x62), UDSStruct.DataIdentifier, uint16(UDSStruct.pin_engT15));      
       case uint16(0x0757)
          getPosMess(uint8(0x62), UDSStruct.DataIdentifier, uint16(UDSStruct.pin_driveTransPumpVlv));
       case uint16(0x0758)
          getPosMess(uint8(0x62), UDSStruct.DataIdentifier, uint16(UDSStruct.pin_reverseTransPumpVlv));
       case uint16(0x0759)
          getPosMess(uint8(0x62), UDSStruct.DataIdentifier, uint16(UDSStruct.pin_transPumpVlv));
       case uint16(0x075A)
          getPosMess(uint8(0x62), UDSStruct.DataIdentifier, uint16(UDSStruct.pin_techEquipPumpSupply));
       case uint16(0x075B)
          getPosMess(uint8(0x62), UDSStruct.DataIdentifier, uint16(UDSStruct.pin_strAndBrkPumpDistrSupply));
       case uint16(0x075C)
          getPosMess(uint8(0x62), UDSStruct.DataIdentifier, uint16(UDSStruct.pin_spareBrkDistrSupply));
       otherwise
           getNegMess(uint8(0x7F), UDSStruct.Service_id, uint8(0x31));
    end
else 
    getNegMess(uint8(0x7F), UDSStruct.Service_id, uint8(0x31));
end
end

== matlab function VCU_SW/convDIOSttToEnum/MATLAB Function ==
  data: value input; enum output; error input
function enum = convertToDIOStsFcn(value, error)
%#codegen
    if error == uint16(0)
        if value
            enum = StateModeTypes.STT_ENABLE;
        else
            enum = StateModeTypes.STT_DISABLE;
        end
    else
        enum = StateModeTypes.STT_ERROR; 
    end
end

== matlab function VCU_SW/ServerFcn/convDIOStatusTypeToNum/MATLAB Function ==
  data: enum input; value output
function value = convertDIOStsToNumFcn(enum)
%#codegen
    if enum == StatusModeTypes.ON
        value = true;
    else
        value = false;
    end
% for future, if there is error or warning, then set function is not called
end
